simulink model "M_GPS"  (R2022a)
settings: Solver=ode4  StartTime=0.0  StopTime=0.04  FixedStep=0.01  RelTol=1e-3
PreLoadFcn:
  | listing = dir;
  | if (contains([listing .name], 'GPS')) && (contains([listing .name], 'MAP'))
  |     addpath('./GPS', './MAP', './DYN');
  |     addpath( genpath('./MAP') );
  | elseif (contains([listing .name], 'M_GPS.slx'))
  |     addpath('../GPS', '../MAP', '../DYN');
  |     addpath( genpath('../MAP') );
  | else
  | 
  | end
  | 
  | load('BUS_STRUCTURE_GPS.mat');
  | load('BUS_STRUCTURE_DYN.mat');
InitFcn:
  | listing = dir;
  | if (contains([listing .name], 'GPS')) && (contains([listing .name], 'MAP'))
  |     addpath('./GPS', './MAP', './DYN');
  |     addpath( genpath('./MAP') );
  | elseif (contains([listing .name], 'M_GPS.slx'))
  |     addpath('../GPS', '../MAP', '../DYN');
  |     addpath( genpath('../MAP') );
  | else
  | 
  | end
  | 
  | load('BUS_STRUCTURE_GPS.mat');
  | load('BUS_STRUCTURE_DYN.mat');
  | 
  | % Random number seed
  | if ~exist('ranNumSeed', 'var')
  |     ranNumSeed = 2034;
  | end
libraries: sharedtransform x1
settings Model: Creator=ASCL  LastModifiedBy=ASCL
settings DataIOCC: SaveOutput=off  SignalLogging=off  DSMLogging=off  SaveTime=off  ReturnWorkspaceOutputs=off
settings OptimizationCC: BlockReduction=off  DefaultParameterBehavior=Inlined  UseDivisionForNetSlopeComputation=on  GainParamInheritBuiltInType=on  UseFloatMulNetSlope=on  ExpressionFolding=off  PassReuseOutputArgsAs=Individual arguments  ZeroExternalMemoryAtStartup=off  ZeroInternalMemoryAtStartup=off  EfficientFloat2IntCast=on  LifeSpan=inf  OptimizeBlockOrder=speed  DifferentSizesBufferReuse=on  EfficientTunableParamExpr=on
settings DebuggingCC: SignalInfNanChecking=warning  ReadBeforeWriteMsg=EnableAllAsError  WriteAfterWriteMsg=EnableAllAsError  WriteAfterReadMsg=EnableAllAsError  IntegerOverflowMsg=error  ParameterTunabilityLossMsg=error  UniqueDataStoreMsg=error  AssertControl=DisableAll  NonBusSignalsTreatedAsBus=error  SFInvalidInputDataAccessInChartInitDiag=error  SFTransitionOutsideNaturalParentDiag=error  SFUnreachableExecutionPathDiag=error  SFUndirectedBroadcastEventsDiag=error  IntegerSaturationMsg=error
settings HardwareCC: ProdBitPerPointer=32  ProdBitPerSizeT=32  ProdBitPerPtrDiffT=32  ProdLargestAtomicInteger=Long  ProdLargestAtomicFloat=Double  ProdEndianess=BigEndian  ProdWordSize=32  ProdLongLongMode=on  ProdHWDeviceType=Freescale->MPC83xx
settings ModelReferenceCC: ModelReferenceNumInstancesAllowed=Single
settings SFSimCC: CompileTimeRecursionLimit=0  EnableRuntimeRecursion=off  MATLABDynamicMemAlloc=off
settings RTWCC: SystemTargetFile=ert.tlc  TemplateMakefile=ert_default_tmf  GenerateReport=on  RTWUseSimCustomCode=on  BuildConfiguration=Faster Runs  IncludeHyperlinkInReport=on  LaunchReport=on  GenerateTraceInfo=on  GenerateTraceReport=on  GenerateTraceReportSl=on  GenerateTraceReportSf=on  GenerateTraceReportEml=on
settings CodeAppCC: ForceParamTrailComments=on  IgnoreCustomStorageClasses=off  OperatorAnnotations=on  SimulinkDataObjDesc=on  SFDataObjDesc=on  MATLABFcnDesc=on  InsertBlockDesc=on  StateflowObjectComments=on  MATLABSourceComments=on  EnableCustomComments=on  InlinedPrmAccess=Macros  ReqsInCode=on
settings ERTTargetCC: TargetLangStandard=C99 (ISO)  UtilityFuncGeneration=Shared location  GenerateSampleERTMain=on  IncludeMdlTerminateFcn=off  CombineSignalStateStructs=on  SuppressErrorStatus=on  SupportAbsoluteTime=off  SupportNonFinite=off  SupportVariableSizeSignals=on  ParenthesesLevel=Standards  CastingMode=Standards  GenerateSharedConstants=off  InlinedParameterPlacement=NonHierarchical  ERTCustomFileTemplate=example_file_process.tlc  RateTransitionBlockCode=Function  PreserveIfCondition=on  ConvertIfToSwitch=off  EnableSignedLeftShifts=off  EnableSignedRightShifts=off

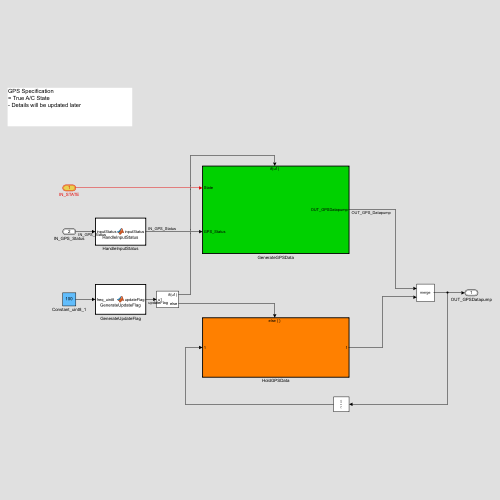
[thumbnail: Simulink's stored preview of the top-level diagram]
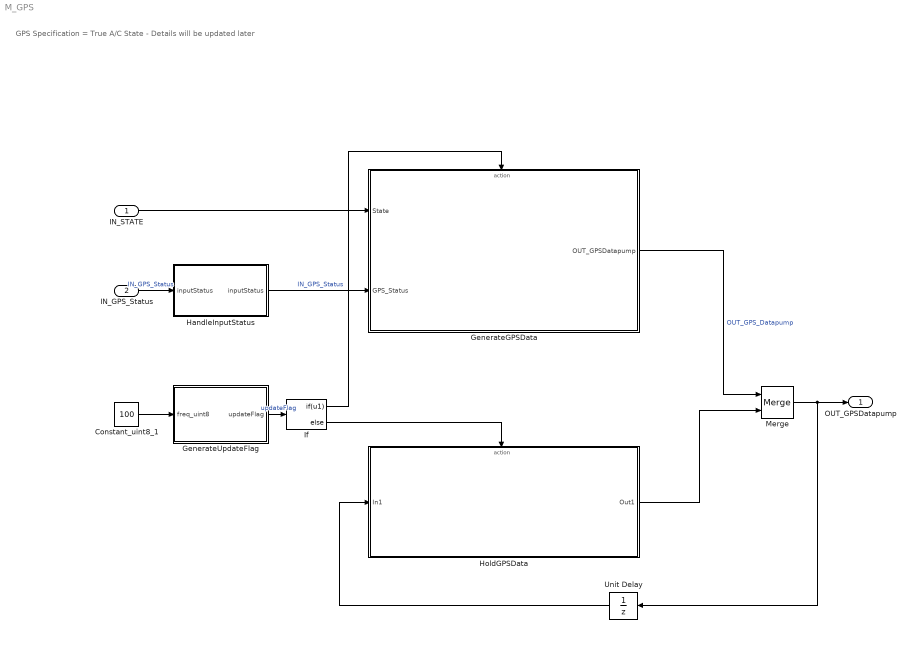
== system M_GPS ==
  note: GPS Specification
      | = True A/C State
      | - Details will be updated later
  IN_STATE : Inport  OutDataTypeStr=Bus: BUS_DYN_STATE  Interpolate=off  BusOutputAsStruct=on
  IN_GPS_Status : Inport  Port=2  OutDataTypeStr=Bus: BUS_SENSOR_GPS_INPUTSTATUS  Interpolate=off  BusOutputAsStruct=on
  Constant_uint8_1 : Constant  Value=100  OutDataTypeStr=uint8
  GenerateGPSData : Subsystem
  GenerateUpdateFlag : MATLAB Function  TreatAsAtomicUnit=on  SystemSampleTime=0.01
  HandleInputStatus : MATLAB Function  TreatAsAtomicUnit=on
  HoldGPSData : Subsystem  TreatAsAtomicUnit=on
  If : If  IfExpression=u1
  Merge : Merge
  Unit Delay : UnitDelay  SampleTime=-1  HasFrameUpgradeWarning=on
  OUT_GPSDatapump : Outport  OutDataTypeStr=Bus: BUS_SENSOR_GPS_DP  VectorParamsAs1DForOutWhenUnconnected=off  BusOutputAsStruct=on
  wires:
  IN_STATE/1 -> GenerateGPSData/1(State)
  GenerateGPSData/1(OUT_GPSDatapump) -> Merge/1  "OUT_GPS_Datapump"
  HandleInputStatus/1(inputStatus) -> GenerateGPSData/2(GPS_Status)  "IN_GPS_Status"
  IN_GPS_Status/1 -> HandleInputStatus/1("inputStatus ")  "IN_GPS_Status"
  Constant_uint8_1/1 -> GenerateUpdateFlag/1(freq_uint8)
  GenerateUpdateFlag/1(updateFlag) -> If/1  "updateFlag"
  Merge/1 -> Unit Delay/1, OUT_GPSDatapump/1
  If/1 -> GenerateGPSData/Action
  If/2 -> HoldGPSData/Action
  HoldGPSData/1(Out1) -> Merge/2
  Unit Delay/1 -> HoldGPSData/1(In1)

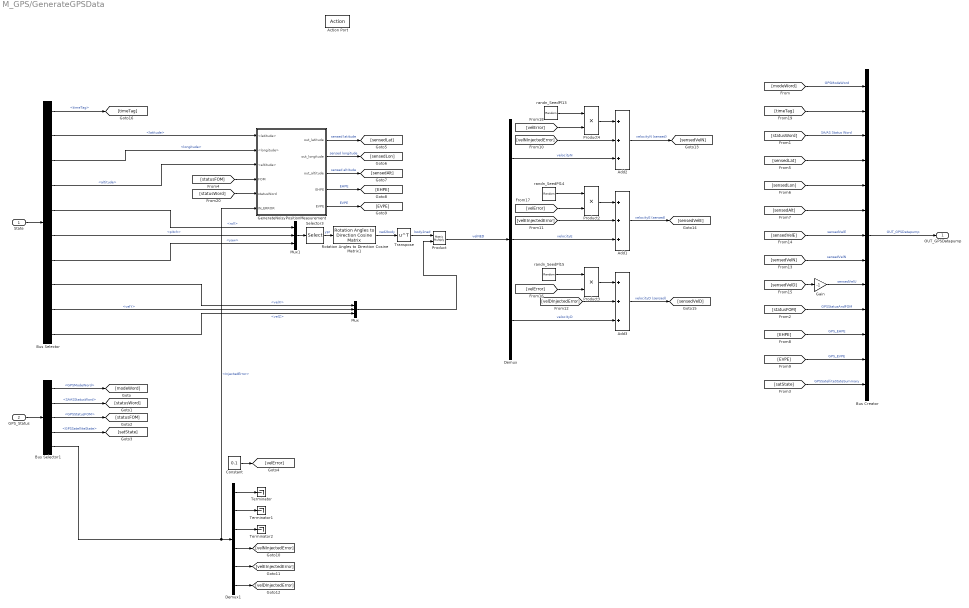
== system M_GPS/GenerateGPSData ==
  State : Inport  OutDataTypeStr=Bus: BUS_DYN_STATE
  GPS_Status : Inport  Port=2  OutDataTypeStr=Bus: BUS_SENSOR_GPS_INPUTSTATUS
  Action Port : ActionPort  ActionPortLabel=if(u1)
  Add1 : Sum  Inputs=+++
  Add2 : Sum  Inputs=+++
  Add3 : Sum  Inputs=+++
  Bus Creator : BusCreator  Inputs=13  OutDataTypeStr=Bus: BUS_SENSOR_GPS_DP  NonVirtualBus=on
      settings: InheritFromInputs=off
  Bus Selector : BusSelector  OutputSignals=timeTag,latitude,longitude,altitude,roll,pitch,yaw,velX,velY,velZ
  Bus Selector1 : BusSelector  OutputSignals=GPSModeWord,SAASStatusWord,GPSStatusFOM,GPSSatelliteState,InjectedError
  Constant : Constant  Value=0.1
  Demux : Demux  Outputs=3
  Demux1 : Demux  Outputs=6
  Gain : Gain  Gain=-1
  GenerateNoisyPositionMeasurement : Subsystem
  Mux : Mux  Inputs=3
  Mux1 : Mux  Inputs=3
  Product : Product  Multiplication=Matrix(*)
  Product2 : Product
  Product3 : Product
  Product4 : Product
  Rotation Angles to Direction Cosine Matrix1 : sharedtransform/Rotation Angles to Direction Cosine Matrix  rotationOrder=ZYX  aMode=aMode
      settings: SourceProductBaseCode=AE,PW,DR,MT,VE
  Selector3 : Selector  IndexMode=Zero-based  InputPortWidth=3  IndexOptions=Index vector (dialog)  Indices=[2 1 0]  OutputSizes=1
  Terminator : Terminator
  Terminator1 : Terminator
  Terminator2 : Terminator
  Transpose : Math  Operator=transpose
  randn_SeedPl13 : RandomNumber  Seed=(ranNumSeed+13)  SampleTime=0.01
  randn_SeedPl14 : RandomNumber  Seed=(ranNumSeed+14)  SampleTime=0.01
  randn_SeedPl15 : RandomNumber  Seed=(ranNumSeed+15)  SampleTime=0.01
  OUT_GPSDatapump : Outport  OutDataTypeStr=Bus: BUS_SENSOR_GPS_DP
  wires:
  [statusWord] -> Bus Creator/3  "SA/AS Status Word"
  [statusFOM] -> Bus Creator/10  "GPSStatusAndFOM"
  Bus Selector/1 -> [timeTag]  "<timeTag>"
  [satState] -> Bus Creator/13  "GPSSatelliteStateSummary"
  [modeWord] -> Bus Creator/1  "GPSModeWord"
  Bus Selector/2 -> GenerateNoisyPositionMeasurement/1(<latitude>)  "<latitude>"
  Bus Selector/10 -> Mux/3  "<velZ>"
  Bus Selector/4 -> GenerateNoisyPositionMeasurement/3(<altitude>)  "<altitude>"
  Bus Selector/3 -> GenerateNoisyPositionMeasurement/2(<longitude>)  "<longitude>"
  State/1 -> Bus Selector/1
  Bus Selector/9 -> Mux/2  "<velY>"
  Bus Selector/8 -> Mux/1  "<velX>"
  Selector3/1 -> Rotation Angles to Direction Cosine Matrix1/1  "ypr"
  Bus Selector/6 -> Mux1/2  "<pitch>"
  Bus Selector/5 -> Mux1/1  "<roll>"
  Bus Selector/7 -> Mux1/3  "<yaw>"
  Mux1/1 -> Selector3/1
  Rotation Angles to Direction Cosine Matrix1/1 -> Transpose/1  "ned2body"
  Transpose/1 -> Product/1  "body2ned"
  Mux/1 -> Product/2
  Product/1 -> Demux/1  "velNED"
  GPS_Status/1 -> Bus Selector1/1
  Bus Selector1/1 -> [modeWord]  "<GPSModeWord>"
  Bus Selector1/2 -> [statusWord]  "<SAASStatusWord>"
  Bus Selector1/3 -> [statusFOM]  "<GPSStatusFOM>"
  Bus Selector1/4 -> [satState]  "<GPSSatelliteState>"
  Bus Selector1/5 -> Demux1/1, GenerateNoisyPositionMeasurement/6(IN_ERROR)  "<InjectedError>"
  [statusFOM] -> GenerateNoisyPositionMeasurement/4(FOM)
  GenerateNoisyPositionMeasurement/1(out_latitude) -> [sensedLat]  "sensed latitude"
  GenerateNoisyPositionMeasurement/2(out_longitude) -> [sensedLon]  "sensed longitude"
  GenerateNoisyPositionMeasurement/3(out_altitude) -> [sensedAlt]  "sensed altitude"
  GenerateNoisyPositionMeasurement/5(EVPE) -> [EVPE]  "EVPE"
  GenerateNoisyPositionMeasurement/4(EHPE) -> [EHPE]  "EHPE"
  randn_SeedPl13/1 -> Product4/1
  [velError] -> Product4/2
  Add2/1 -> [sensedVelN]  "velocityN (sensed)"
  [velError] -> Product2/2
  randn_SeedPl14/1 -> Product2/1
  randn_SeedPl15/1 -> Product3/1
  [velError] -> Product3/2
  Product3/1 -> Add3/1
  Demux/3 -> Add3/3  "velocityD"
  Add1/1 -> [sensedVelE]  "velocityE (sensed)"
  Add3/1 -> [sensedVelD]  "velocityD (sensed)"
  Demux1/3 -> Terminator2/1
  Demux1/2 -> Terminator1/1
  Demux1/1 -> Terminator/1
  Demux1/4 -> [velNInjectedError]
  Demux1/5 -> [velEInjectedError]
  Demux1/6 -> [velDInjectedError]
  [velDInjectedError] -> Add3/2
  [sensedLat] -> Bus Creator/4
  [sensedLon] -> Bus Creator/5
  [sensedAlt] -> Bus Creator/6
  Gain/1 -> Bus Creator/9  "sensedVelU"
  [sensedVelD] -> Gain/1
  [sensedVelN] -> Bus Creator/8  "sensedVelN"
  [sensedVelE] -> Bus Creator/7  "sensedVelE"
  [EHPE] -> Bus Creator/11  "GPS_EHPE"
  [EVPE] -> Bus Creator/12  "GPS_EVPE"
  Bus Creator/1 -> OUT_GPSDatapump/1  "OUT_GPSDatapump"
  Demux/2 -> Add1/3  "velocityE"
  Product2/1 -> Add1/1
  Product4/1 -> Add2/1
  Demux/1 -> Add2/3  "velocityN"
  [velNInjectedError] -> Add2/2
  [velEInjectedError] -> Add1/2
  [timeTag] -> Bus Creator/2
  [statusWord] -> GenerateNoisyPositionMeasurement/5(statusWord)
  Constant/1 -> [velError]

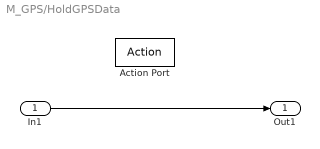
== system M_GPS/HoldGPSData ==
  In1 : Inport
  Action Port : ActionPort  ActionPortLabel=else
  Out1 : Outport
  wires:
  In1/1 -> Out1/1

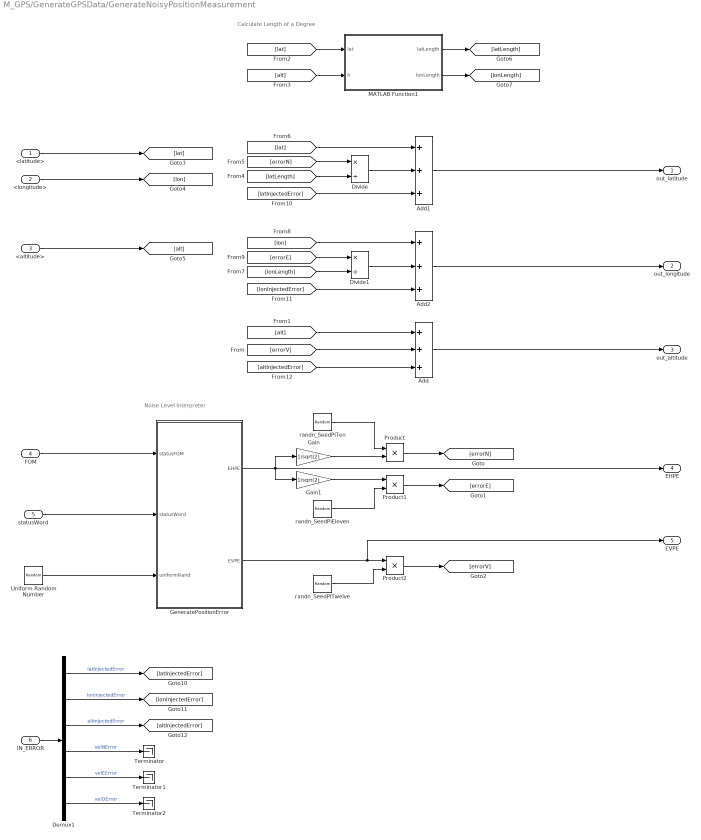
== system M_GPS/GenerateGPSData/GenerateNoisyPositionMeasurement ==
  note: Noise Level Interpreter
  note: Calculate Length of a Degree
  <latitude> : Inport
  <longitude> : Inport  Port=2
  <altitude> : Inport  Port=3
  FOM : Inport  Port=4
  statusWord : Inport  Port=5
  IN_ERROR : Inport  Port=6
  Add : Sum  Inputs=+++
  Add1 : Sum  Inputs=+++
  Add2 : Sum  Inputs=+++
  Demux1 : Demux  Outputs=6
  Divide : Product  Inputs=*/
  Divide1 : Product  Inputs=*/
  Gain : Gain  Gain=1/sqrt(2)
  Gain1 : Gain  Gain=1/sqrt(2)
  GeneratePositionError : MATLAB Function  TreatAsAtomicUnit=on  SystemSampleTime=0.01
  MATLAB Function1 : MATLAB Function  TreatAsAtomicUnit=on
  Product : Product
  Product1 : Product
  Product2 : Product
  Terminator : Terminator
  Terminator1 : Terminator
  Terminator2 : Terminator
  Uniform Random Number : UniformRandomNumber  Minimum=0  Seed=ranNumSeed  SampleTime=0.01
  randn_SeedPlEleven : RandomNumber  Seed=(ranNumSeed+11)  SampleTime=0.01
  randn_SeedPlTen : RandomNumber  Seed=(ranNumSeed+10)  SampleTime=0.01
  randn_SeedPlTwelve : RandomNumber  Seed=(ranNumSeed+12)  SampleTime=0.01
  out_latitude : Outport
  out_longitude : Outport  Port=2
  out_altitude : Outport  Port=3
  EHPE : Outport  Port=4
  EVPE : Outport  Port=5
  wires:
  <latitude>/1 -> [lat]
  FOM/1 -> GeneratePositionError/1(statusFOM)
  GeneratePositionError/1(EHPE) -> EHPE/1, Gain1/1, Gain/1
  randn_SeedPlTen/1 -> Product/1
  Gain/1 -> Product/2
  Gain1/1 -> Product1/1
  randn_SeedPlEleven/1 -> Product1/2
  GeneratePositionError/2(EVPE) -> EVPE/1, Product2/1
  randn_SeedPlTwelve/1 -> Product2/2
  Product/1 -> [errorN]
  Product1/1 -> [errorE]
  Product2/1 -> [errorV]
  [errorV] -> Add/2
  <altitude>/1 -> [alt]
  Add/1 -> out_altitude/1
  <longitude>/1 -> [lon]
  [alt] -> Add/1
  [lat] -> MATLAB Function1/1(lat)
  [alt] -> MATLAB Function1/2(h)
  MATLAB Function1/1(latLength) -> [latLength]
  MATLAB Function1/2(lonLength) -> [lonLength]
  [latLength] -> Divide/2
  [errorN] -> Divide/1
  [lat] -> Add1/1
  Divide/1 -> Add1/2
  Add1/1 -> out_latitude/1
  Add2/1 -> out_longitude/1
  [lonLength] -> Divide1/2
  [lon] -> Add2/1
  [errorE] -> Divide1/1
  Divide1/1 -> Add2/2
  Demux1/3 -> [altInjectedError]  "altInjectedError"
  Demux1/1 -> [latInjectedError]  "latInjectedError"
  Demux1/4 -> Terminator/1  "velNError"
  Demux1/2 -> [lonInjectedError]  "lonInjectedError"
  Demux1/5 -> Terminator1/1  "velEError"
  Demux1/6 -> Terminator2/1  "velDError"
  IN_ERROR/1 -> Demux1/1
  [latInjectedError] -> Add1/3
  [lonInjectedError] -> Add2/3
  [altInjectedError] -> Add/3
  statusWord/1 -> GeneratePositionError/2(statusWord)
  Uniform Random Number/1 -> GeneratePositionError/3(uniformRand)

== matlab function M_GPS/GenerateGPSData/GenerateNoisyPositionMeasurement/MATLAB Function1 ==
  data: lat input; latLength output; h input; lonLength output
function [latLength, lonLength] = getLengthOfADegree(lat, h)
%GETLENGTHOFADEGREE
% Calculate the length of one degree of both latitude and longitude
% for a specified latitude and height
%
% == Inputs =========
% lat               - Latitude [deg]
% h                 - Height [m]
% 
% == Outputs ========
% latLength         - Length of 1 deg of latitude on the ref. spheroid [m]
% lonLength         - Length of 1 deg of longitude on the ref. spheroid [m]
% ===================
%%%%%%%%%%%%%%%%%%%%%%%%%%%%%%%%%%%%%%%%%%%%%%%%%%%%%%%%%%%%%%%%%%%%%%%%%%%

if nargin < 2
    h   = 0.0;
end

% WGS84 Parameters
eRadius = 6378137.0;
eEccen = 0.08181919;

% Radius of curvature in prime vertical
nE = eRadius / sqrt( 1 - (eEccen^2*(sind(lat))^2) );
% Meridian Radius of Curavature
mE = eRadius * (1 - eEccen^2) / (1 - eEccen^2*(sind(lat))^2)^(1.5);

lonLength = (nE + h) * cosd(lat) * (pi/180);
latLength = (mE + h) * (pi/180);

end

== matlab function M_GPS/GenerateGPSData/GenerateNoisyPositionMeasurement/GeneratePositionError ==
  data: statusFOM input; EHPE output; EVPE output; statusWord input; uniformRand input
function [EHPE, EVPE] = GeneratePositionError(statusFOM, statusWord, uniformRand)
%GeneratePositionError

%
persistent variableNoise count
if isempty(variableNoise)
    variableNoise = uniformRand;
end
if isempty(count)
    count = uint32(0);
end

if (count == uint32(0))
    variableNoise = uniformRand;
    variableNoise = max(0, min(1, variableNoise)); % saturate on [0, 1]
end

% Initialize
EHPE = 0;
EVPE = 0;

PCodeAvailable = logical(bitget(statusWord, 1)); 
% FOM = bitget(statusFOM, 13) + uint16(2) * bitget(statusFOM, 14) + uint16(4) * bitget(statusFOM, 15) + uint16(8) * bitget(statusFOM, 16);
FOM = statusFOM;
if (PCodeAvailable)

    EPE = 6.25 + 4.3 * variableNoise;

else
    switch FOM
        case uint16(1)
            EPE = 12.5 + 12.5 * variableNoise;

        case uint16(2)
            EPE = 25 + 25 * variableNoise;

        case uint16(3)
            EPE = 50 + 25 * variableNoise;

        case uint16(4)
            EPE = 75 + 25 * variableNoise;

        case uint16(5)
            EPE = 100 + 100 * variableNoise;

        case uint16(6)
            EPE = 200 + 300 * variableNoise;

        case uint16(7)
            EPE = 500 + 500 * variableNoise;

        case uint16(8)
            EPE = 1000 + 4000 * variableNoise;

        case uint16(9)
            EPE = 5000 + 4000 * variableNoise;

        otherwise
            EPE = 0 + 25 * variableNoise;
    end
end

EHPE = 1.1851/sqrt(5) * EPE;
EVPE = 1.8962/sqrt(5) * EPE;

count = count + uint32(1);
if (count > uint32(1000))
    count = uint32(0);
end
 
end


%%
% REFERENCE
% GPS FORM related to EPE
% -----------------------
%  FOM       EPE(m) 1-sigma RMSE
% -----------------------
%   1       < 25
%   2       < 50
%   3       < 75
%   4       < 100
%   5       < 200
%   6       < 500
%   7       < 1,000
%   8       < 5,000
%   9       > 5,000

== matlab function M_GPS/GenerateUpdateFlag ==
  settings: updateMethod=DISCRETE  sampleTime=0.01
  data: updateFlag output boolean; freq_uint8 input uint8
function updateFlag = GenerateUpdateFlag(freq_uint8)
%GenerateUpdateFlag RALT 데이터 갱신 플래그 생성
% Input
% - freq_uint8  1 = update data at every simulation step
%               25 = update data at every 25 simulation steps
%               Accepts  (8bit unsigned integer=uint8) only
% Output
% - updateFlag  True/False
persistent cnt

assert (isa(freq_uint8, 'uint8'))

if isempty(cnt)
    cnt = uint8(0);
end

% Initialize
updateFlag = false;

if mod(cnt, freq_uint8) == uint8(0)
    updateFlag = true;
    cnt = uint8(1);
else
    updateFlag = false;
    cnt = cnt + uint8(1);
end

end

== matlab function M_GPS/HandleInputStatus ==
  data: inputStatus input Bus: BUS_SENSOR_GPS_INPUTSTATUS; inputStatus output
function inputStatus = HandleInputStatus(inputStatus)

if(inputStatus.InputActivated)
    
else
    inputStatus.GPSModeWord         = uint16(0b0000000000000001); % NavData valid
    inputStatus.SAASStatusWord      = uint16(0b0000000000000001); % P code
    inputStatus.GPSStatusFOM        = uint16(1); % FOM = 1
%     inputStatus.GPSStatusFOM        = uint16(2); % FOM = 2
%     inputStatus.GPSStatusFOM        = uint16(3); % FOM = 3
%     inputStatus.GPSStatusFOM        = uint16(4); % FOM = 4
%     inputStatus.GPSStatusFOM        = uint16(5); % FOM = 5
%     inputStatus.GPSStatusFOM        = uint16(6); % FOM = 6
    inputStatus.GPSSatelliteState   = uint16(0b0000000000000001); % No of ch.
end
